simulink model "sampleModel1680"  (R2023a)
settings: Solver=VariableStepAuto  StartTime=0.0  StopTime=10.0  RelTol=1e-3
libraries: hdlsllib x6, simulink x2
settings Model: Creator=user1  LastModifiedBy=user1

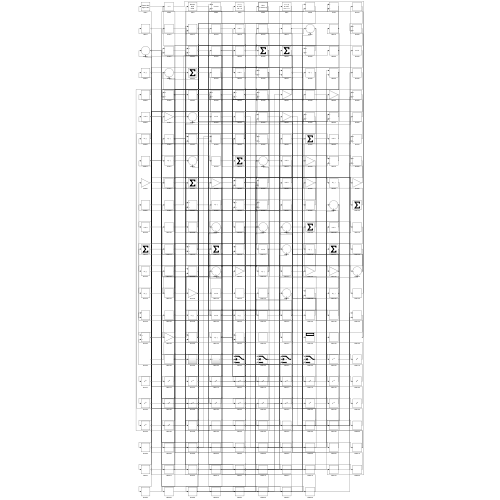
[thumbnail: Simulink's stored preview of the top-level diagram]
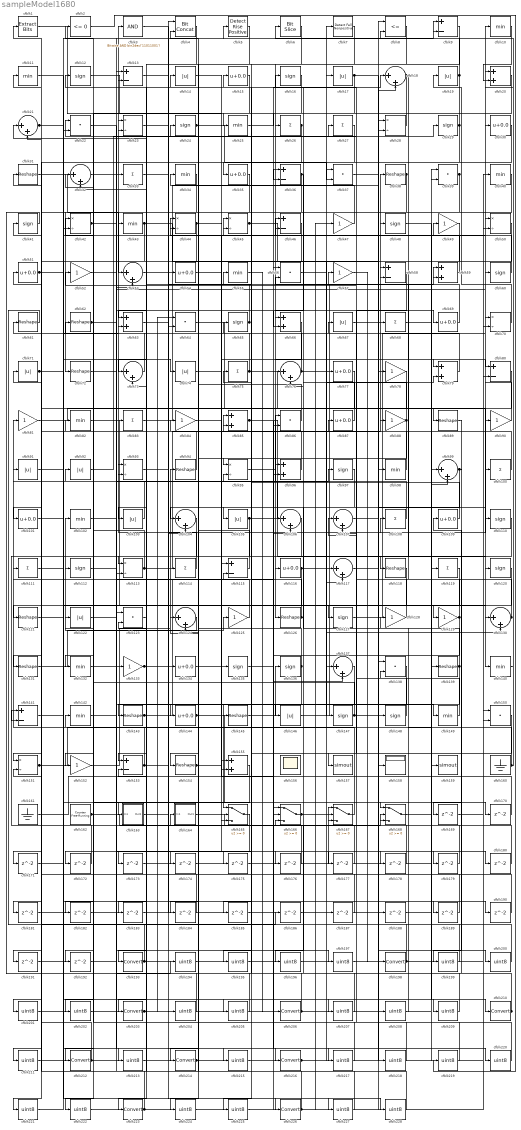
== system sampleModel1680 ==
  cfblk1 : simulink/Logic and Bit Operations/Extract Bits  bitsToExtract=Upper half  numBits=8  bitIdxRange=[0 7]  outScalingMode=Preserve fixed-point scaling
      settings: LibrarySourceBlock=|
      | hdlsllib/Logic and Bit
      | Operations/Extract Bits
  cfblk{10..11,25,34,40,43,55,82,98,102,132,140,142,149} (14 alike) : MinMax
  cfblk{26..27,33,68,75,83,100,108,111,114,119} (11 alike) : Sum  Inputs=+
  cfblk{15,30,35,51,54,69,77,87,101,109,116,134,144} (13 alike) : Bias  Bias=0.0  SaturateOnIntegerOverflow=off
  cfblk{14,17,19,67,71,74,91..92,103,105,122,146} (12 alike) : Abs  SaturateOnIntegerOverflow=off
  cfblk{18,21,32,53,73,76,99,104,106..107,117,124,130,137} (14 alike) : Sum  Inputs=|++
  cfblk{12,16,24,29,41,48,60,65,97,110,112,120,127,135..136,147..148} (17 alike) : Signum
  cfblk{23,28,42,44..45,50,70,93,95,113,151} (11 alike) : Product  Inputs=*/  RndMeth=Zero  SaturateOnIntegerOverflow=on
  cfblk{9,13,36,46,58,80,115,141,153} (9 alike) : Sum  Inputs=+-
  cfblk{31,38,61..62,72,89,94,118,121,126,131,139,143,145,154} (15 alike) : Reshape
  cfblk{22,37,39,56,64,86,123,138,150} (9 alike) : DotProduct  OutDataTypeStr=Inherit: Inherit via internal rule
  cfblk{47,49,52,57,78,81,84,88,90,125,128..129,133,152} (14 alike) : Gain
  cfblk{20,59,63,66,79,85,96,155} (8 alike) : Sum
  cfblk156 : Scope
      settings: Floating=on
  cfblk157 : ToWorkspace  VariableName=simout  SaveFormat=Timeseries  SampleTime=-1
  cfblk158 : Display
  cfblk159 : ToWorkspace  VariableName=simout  SaveFormat=Timeseries  SampleTime=-1
  cfblk160 : Ground
  cfblk161 : Ground
  cfblk162 : hdlsllib/Sources/Counter Free-Running  NumBits=16  tsamp=-1
  cfblk163 : Subsystem
      settings: LibrarySourceBlock=|
      | hdlsllib/Ports &
      | Subsystems/Subsystem
  cfblk164 : Subsystem
      settings: LibrarySourceBlock=|
      | hdlsllib/Ports &
      | Subsystems/Subsystem
  cfblk{165..168} (4 alike) : Switch  SaturateOnIntegerOverflow=off  InputSameDT=off
  cfblk{169..192} (24 alike) : Delay  SampleTime=1
  cfblk{193,198,203,206,210,212,214,216,223,226} (10 alike) : DataTypeConversion  SaturateOnIntegerOverflow=off  RndMeth=Floor
  cfblk{194..197,199..202,204..205,207..209,211,213,215,217..222,224..225,227..228} (26 alike) : DataTypeConversion  OutDataTypeStr=uint8  SaturateOnIntegerOverflow=off  RndMeth=Floor
  cfblk2 : hdlsllib/Logic and Bit Operations/Compare To Zero  relop=<=  OutDataTypeStr=boolean
  cfblk3 : simulink/Logic and Bit Operations/Bitwise Operator  logicop=AND  UseBitMask=on  BitMask=bin2dec('11011001')  BitMaskRealWorld=Stored Integer
      settings: LibrarySourceBlock=|
      | hdlsllib/Logic and Bit
      | Operations/Bitwise
      | Operator
  cfblk4 : hdlsllib/Logic and Bit Operations/Bit Concat  numInputs=2
  cfblk5 : hdlsllib/Logic and Bit Operations/Detect Rise Positive  vinit=0  OutDataTypeStr=boolean
  cfblk6 : hdlsllib/Logic and Bit Operations/Bit Slice  lidx=7  ridx=0
  cfblk7 : hdlsllib/Logic and Bit Operations/Detect Fall Nonpositive  vinit=0  OutDataTypeStr=boolean
  cfblk8 : RelationalOperator  Operator=<=  OutDataTypeStr=boolean  InputSameDT=off
  wires:
  cfblk153/1 -> cfblk81/1, cfblk95/2
  cfblk113/1 -> cfblk85/1, cfblk42/1
  cfblk64/1 -> cfblk140/1
  cfblk140/1 -> cfblk6/1
  cfblk36/1 -> cfblk66/1, cfblk42/2, cfblk171/1
  cfblk138/1 -> cfblk165/1
  cfblk124/1 -> cfblk102/1
  cfblk145/1 -> cfblk136/1
  cfblk90/1 -> cfblk10/1
  cfblk92/1 -> cfblk29/1
  cfblk132/1 -> cfblk94/1
  cfblk162/1 -> cfblk167/1, cfblk60/1
  cfblk9/1 -> cfblk126/1
  cfblk42/1 -> cfblk66/2, cfblk217/1
  cfblk126/1 -> cfblk75/1, cfblk76/2
  cfblk141/1 -> cfblk9/1
  cfblk109/1 -> cfblk45/1
  cfblk85/1 -> cfblk120/1, cfblk209/1
  cfblk106/1 -> cfblk223/1
  cfblk114/1 -> cfblk3/1
  cfblk115/1 -> cfblk23/1
  cfblk28/1 -> cfblk26/1
  cfblk68/1 -> cfblk210/1
  cfblk34/1 -> cfblk72/1
  cfblk47/1 -> cfblk34/1
  cfblk129/1 -> cfblk22/1, cfblk166/2, cfblk87/1
  cfblk39/1 -> cfblk53/1, cfblk192/1
  cfblk136/1 -> cfblk111/1, cfblk174/1
  cfblk93/1 -> cfblk59/1
  cfblk144/1 -> cfblk168/1, cfblk48/1
  cfblk66/1 -> cfblk116/1
  cfblk116/1 -> cfblk38/1, cfblk184/1, cfblk185/1
  cfblk147/1 -> cfblk8/1, cfblk32/1
  cfblk84/1 -> cfblk49/1
  cfblk82/1 -> cfblk166/1
  cfblk83/1 -> cfblk28/1
  cfblk96/1 -> cfblk65/1
  cfblk146/1 -> cfblk30/1
  cfblk4/1 -> cfblk103/1
  cfblk79/1 -> cfblk15/1
  cfblk33/1 -> cfblk146/1
  cfblk52/1 -> cfblk8/2
  cfblk77/1 -> cfblk214/1
  cfblk13/1 -> cfblk226/1
  cfblk58/1 -> cfblk157/1
  cfblk24/1 -> cfblk37/2, cfblk79/1
  cfblk56/1 -> cfblk130/1
  cfblk30/1 -> cfblk35/1
  cfblk100/1 -> cfblk41/1
  cfblk152/1 -> cfblk114/1
  cfblk95/1 -> cfblk86/1
  cfblk125/1 -> cfblk14/1
  cfblk119/1 -> cfblk143/1
  cfblk122/1 -> cfblk149/1
  cfblk127/1 -> cfblk70/1
  cfblk49/1 -> cfblk95/1
  cfblk18/1 -> cfblk113/1, cfblk118/1
  cfblk50/1 -> cfblk101/1
  cfblk70/1 -> cfblk19/1
  cfblk86/1 -> cfblk24/1
  cfblk29/1 -> cfblk25/1, cfblk73/2
  cfblk142/1 -> cfblk216/1
  cfblk6/1 -> cfblk105/1
  cfblk75/1 -> cfblk100/1, cfblk44/2
  cfblk151/1 -> cfblk99/1, cfblk46/2
  cfblk81/1 -> cfblk89/1
  cfblk73/1 -> cfblk11/1
  cfblk130/1 -> cfblk52/1, cfblk58/2
  cfblk160/1 -> cfblk20/1, cfblk138/2
  cfblk21/1 -> cfblk165/3, cfblk207/1
  cfblk120/1 -> cfblk163/1(In1)
  cfblk8/1 -> cfblk154/1
  cfblk131/1 -> cfblk125/1
  cfblk72/1 -> cfblk33/1
  cfblk37/1 -> cfblk98/1
  cfblk143/1 -> cfblk56/1, cfblk108/1
  cfblk103/1 -> cfblk62/1
  cfblk46/1 -> cfblk131/1
  cfblk104/1 -> cfblk151/1
  cfblk164/1(Out1) -> cfblk168/2
  cfblk133/1 -> cfblk4/1, cfblk93/2
  cfblk62/1 -> cfblk113/2, cfblk90/1
  cfblk148/1 -> cfblk93/1
  cfblk69/1 -> cfblk56/2
  cfblk94/1 -> cfblk83/1
  cfblk54/1 -> cfblk155/1
  cfblk123/1 -> cfblk203/1
  cfblk45/1 -> cfblk147/1, cfblk175/1
  cfblk135/1 -> cfblk137/2
  cfblk40/1 -> cfblk212/1
  cfblk65/1 -> cfblk21/1, cfblk32/2
  cfblk98/1 -> cfblk58/1
  cfblk60/1 -> cfblk4/2
  cfblk1/1 -> cfblk135/1
  cfblk154/1 -> cfblk88/1, cfblk176/1, cfblk177/1
  cfblk32/1 -> cfblk69/1
  cfblk76/1 -> cfblk2/1, cfblk59/2
  cfblk3/1 -> cfblk54/1
  cfblk110/1 -> cfblk141/2
  cfblk134/1 -> cfblk97/1
  cfblk55/1 -> cfblk206/1
  cfblk31/1 -> cfblk43/1
  cfblk15/1 -> cfblk63/1
  cfblk12/1 -> cfblk134/1
  cfblk87/1 -> cfblk16/1
  cfblk112/1 -> cfblk115/2
  cfblk161/1 -> cfblk86/2
  cfblk137/1 -> cfblk153/1
  cfblk167/1 -> cfblk112/1
  cfblk16/1 -> cfblk73/1
  cfblk71/1 -> cfblk74/1, cfblk181/1, cfblk228/1
  cfblk38/1 -> cfblk145/1, cfblk225/1
  cfblk139/1 -> cfblk155/2, cfblk46/1
  cfblk57/1 -> cfblk198/1
  cfblk80/1 -> cfblk132/1
  cfblk25/1 -> cfblk18/1
  cfblk43/1 -> cfblk158/1, cfblk211/1
  cfblk23/1 -> cfblk127/1
  cfblk108/1 -> cfblk61/1
  cfblk88/1 -> cfblk144/1, cfblk27/1
  cfblk102/1 -> cfblk96/1
  cfblk63/1 -> cfblk5/1
  cfblk118/1 -> cfblk121/1
  cfblk105/1 -> cfblk17/1, cfblk152/1, cfblk224/1
  cfblk168/1 -> cfblk139/1
  cfblk7/1 -> cfblk193/1
  cfblk128/1 -> cfblk82/1
  cfblk19/1 -> cfblk104/1, cfblk9/2
  cfblk51/1 -> cfblk129/1, cfblk190/1
  cfblk44/1 -> cfblk80/1, cfblk191/1
  cfblk17/1 -> cfblk110/1, cfblk36/2
  cfblk74/1 -> cfblk50/1
  cfblk26/1 -> cfblk165/2, cfblk183/1
  cfblk101/1 -> cfblk63/2
  cfblk59/1 -> cfblk44/1
  cfblk10/1 -> cfblk20/2
  cfblk166/1 -> cfblk130/2, cfblk79/2
  cfblk149/1 -> cfblk12/1
  cfblk99/1 -> cfblk124/2, cfblk169/1
  cfblk169/1 -> cfblk70/2
  cfblk91/1 -> cfblk170/1
  cfblk170/1 -> cfblk115/1
  cfblk35/1 -> cfblk172/1
  cfblk172/1 -> cfblk141/1
  cfblk5/1 -> cfblk173/1
  cfblk173/1 -> cfblk167/3
  cfblk174/1 -> cfblk96/2
  cfblk175/1 -> cfblk99/2
  cfblk176/1 -> cfblk85/2
  cfblk177/1 -> cfblk153/2
  cfblk22/1 -> cfblk178/1
  cfblk178/1 -> cfblk1/1
  cfblk14/1 -> cfblk179/1
  cfblk179/1 -> cfblk168/3
  cfblk48/1 -> cfblk180/1
  cfblk180/1 -> cfblk45/2
  cfblk181/1 -> cfblk64/2
  cfblk165/1 -> cfblk182/1
  cfblk182/1 -> cfblk18/2
  cfblk183/1 -> cfblk104/2
  cfblk184/1 -> cfblk21/2
  cfblk61/1 -> cfblk186/1
  cfblk186/1 -> cfblk137/1
  cfblk187/1 -> cfblk151/2
  cfblk188/1 -> cfblk39/2
  cfblk11/1 -> cfblk189/1
  cfblk189/1 -> cfblk23/2
  cfblk190/1 -> cfblk124/1
  cfblk191/1 -> cfblk53/2
  cfblk193/1 -> cfblk50/2, cfblk76/1, cfblk91/1
  cfblk41/1 -> cfblk194/1
  cfblk194/1 -> cfblk7/1
  cfblk150/1 -> cfblk195/1
  cfblk195/1 -> cfblk167/2
  cfblk97/1 -> cfblk196/1
  cfblk196/1 -> cfblk150/1
  cfblk192/1 -> cfblk197/1
  cfblk197/1 -> cfblk150/2
  cfblk198/1 -> cfblk138/1, cfblk122/1
  cfblk89/1 -> cfblk199/1
  cfblk199/1 -> cfblk57/1
  cfblk117/1 -> cfblk200/1
  cfblk200/1 -> cfblk71/1
  cfblk27/1 -> cfblk201/1
  cfblk201/1 -> cfblk117/1
  cfblk20/1 -> cfblk202/1
  cfblk202/1 -> cfblk117/2
  cfblk203/1 -> cfblk159/1, cfblk64/1
  cfblk53/1 -> cfblk204/1
  cfblk204/1 -> cfblk123/1
  cfblk171/1 -> cfblk205/1
  cfblk205/1 -> cfblk123/2
  cfblk206/1 -> cfblk148/1, cfblk164/1(In1), cfblk39/1
  cfblk207/1 -> cfblk55/1
  cfblk67/1 -> cfblk208/1
  cfblk208/1 -> cfblk128/1
  cfblk209/1 -> cfblk67/1
  cfblk210/1 -> cfblk166/3, cfblk109/1
  cfblk211/1 -> cfblk68/1
  cfblk212/1 -> cfblk133/1, cfblk51/1
  cfblk121/1 -> cfblk213/1
  cfblk213/1 -> cfblk40/1
  cfblk214/1 -> cfblk36/1, cfblk37/1
  cfblk163/1(Out1) -> cfblk215/1
  cfblk215/1 -> cfblk77/1
  cfblk216/1 -> cfblk188/1, cfblk187/1, cfblk119/1
  cfblk217/1 -> cfblk142/1
  cfblk107/1 -> cfblk218/1
  cfblk218/1 -> cfblk92/1
  cfblk2/1 -> cfblk219/1
  cfblk219/1 -> cfblk107/1
  cfblk185/1 -> cfblk220/1
  cfblk220/1 -> cfblk107/2
  cfblk78/1 -> cfblk221/1
  cfblk221/1 -> cfblk22/2
  cfblk155/1 -> cfblk222/1
  cfblk222/1 -> cfblk78/1
  cfblk223/1 -> cfblk28/2, cfblk80/2, cfblk31/1
  cfblk224/1 -> cfblk106/1
  cfblk225/1 -> cfblk106/2
  cfblk226/1 -> cfblk84/1, cfblk47/1
  cfblk111/1 -> cfblk227/1
  cfblk227/1 -> cfblk13/1
  cfblk228/1 -> cfblk13/2

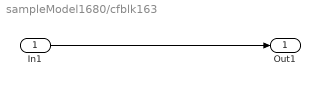
== system sampleModel1680/cfblk163 ==
  In1 : Inport
  Out1 : Outport
  wires:
  In1/1 -> Out1/1

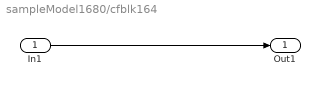
== system sampleModel1680/cfblk164 ==
  In1 : Inport
  Out1 : Outport
  wires:
  In1/1 -> Out1/1
